simulink subsystem "PvtSubSys_HMI"  (R2020b)
settings: Solver=VariableStepAuto  StartTime=0.0  StopTime=10.0  RelTol=1e-3
undefined symbols (not defined in the file): P_HMI_LDW_LKAWarnTime, P_HMI_ObjectTypeFilter, P_HMI_WarnFormLDWReq
libraries: simulink x212, TrueDurationTime x6
(part 1 of 8)
settings Model: Creator=GW00133806  LastModifiedBy=GW00201299

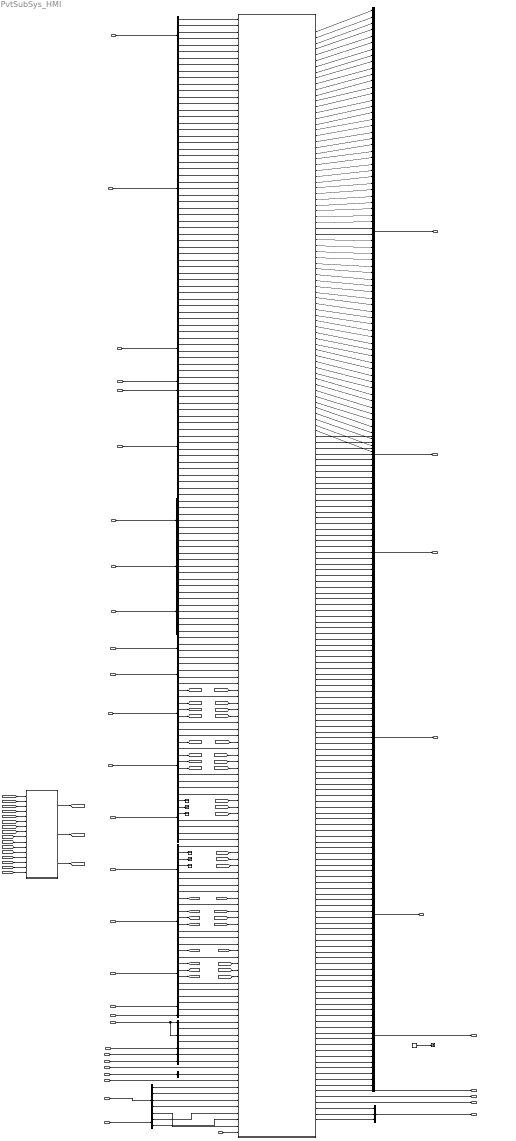
== system PvtSubSys_HMI ==
  note: HMI变更历史
      | Author:XTY
      | Version:HMI_V1.0
      | Data:2020/9/18
      | Description:
      | 可删除信号：
      |              输入：LONC_ACC_TakeOverReq；
      |                         LONC_IntelligentCurveActive；
      |              输出：Longctrl_HCUTrqReq_DVR；
      |                         ACC_TakeOverReq
      |                         Longctrl_HCUTrqReqActive_DVR
      |                         IntelligentCurveAct
      |
      | Data:2020/10/31
      | Description:
      | IFC_Signal模块：
      |                （1）增加了ELK状态显示策略
      |                （2）增加了ESS状态显示策略
      |
      | Data:2020/11/03
      | Description:
      | IFC_Signal模块：
      |                (1)增加了ELK和LCK/LKA互动关系逻辑；
      | 修正LSSErrSts逻辑；
      |                (2)增加了LSSSwt总开关逻辑；只有在LSSSwt打
      | 开的情况下，才能在3L功能任选其一；
      |                (3)增加了LCKIESts信号；方便HUT开关逻辑编写；
      |                                                                           ——2020/11/03
      |
      | Data:2020/11/05
      | Description:
      | HWA/ACC/TJA_Signal模块：
      | 1）临时增加了HWA的退出报警；
      | 11/11:
      | 增加了ACC/TJA/HWA文字提示的信号延时发送3s；
      |
      | Data:2020/11/13
      | Description:
      | （1）LDW_LKAWarn该信号接地
      | （2）释放AES输出信号：
      |           AESResp；AESSts；AESErrSts; AESintervention
      | （3）连上ACC_TakeOver；by hu；
      |
      | 2020/11/14
      | 1)ACC/TJA/HWA文字提醒调整；
      | 2)增加HMI模块的counter；
      |
      | 2020/11/19
      | 1)ACC目标显示梳理；
      | 2)HWAWarning时不报HandsOffWarning；
      |
      | 2020/11/23
      | 1)删除ACC_DataRecReq；
      | 2)HWAWarning，HandsOffWarning，DriverSts三者交互逻辑调整。
      |
      | 2020/11/30
      | （1） 增加了L1blsLineExist/ R1blsLineExist 两个信号；
      | 用来计算IFC_LaneCurve；
      | （2）关联TJAState与LSSIntervention；
      | （3）关联LSS_WarnFormSwtReq与LSSIntervention；
      | （4）增加LSSSwtReq 信号的“软开关”；修改横向功能
      | 输出；
      | （5）增加了LDW_LKAWarn信号输出
      | （6）增加了F_LBblsLineExist和F_RBblsLineExist两条
      | 边界有效性信号，用于输出计算仪表车道线信息；
      |
      | 2020/12/02
      | （1）IFCvibrationwarning信号关联LSSInTervention信号
      | only reminder coding值；
      | （2）关联TJAState与LSSIntervention及其横向状态；
      |
      | 2020/12/03
      | （1）添加了LCKSwtReq 信号；
      | （2）添加了标定量P_HMI_LDW_LKAWarnTime；
      | (3)连上ACC目标p4和p5的有效性和类型；
      |
      | 2020/12/11
      | (1)适配NOA新架构；
      | 2020/12/16
      | (1)再次适配NOA新架构，基于新EHR；
      |
      | 2020/12/22
      | 1、基于PLAN和LONG模块更新的架构调整HMI；
      | 2020/12/23
      | 增加distbar输出；
      |
      | 2020.12.29
      | 修改ACC起步提醒信号的发送，输入暂用CCTextDisp，待接口更新；
      | 2021.1.6
      | HWA转向灯请求输出；
      | 2021.1.14
      | 道线的C2,C3增加gain，参考仪表显示文档；
      | 2021.1.21
      | 修改ACC目标显示坐标系，左负右正。
      | 2021.1.27
      | ACC目标HeadingAngle输出单位修改；
      | DrvrSts修改；
      | DriverOffDisp修改；
      | 2021.2.1
      | HMI升级DBC4.1输入接口；
      | 2021.2.3
      | LSSIntervention与TJA对应状态输出修改；
      | 目标显示修改heading修改；
      | fu_type连接；
      | 2021.2.5
      | 道线长度增加12个信号输出；
      | ACCFtSts修改；
      |
      | 2021.2.17
      | 各个线C0的初始值修改；
      | 2021.2.20
      | 增加NOH相关ACC_FD3报文信号；
      | 2021.2.22
      | LCK和ELK和ESS的Error修改；
      | 接口变更增加ACCFD3；
      | HWA_LaneChangeReq修改；
      | 2021.2.25
      | HWA_LaneChangeReq修改。
      | 2021.3.2
      | RoadEdge显示输出修改；
      | 2021.3.4
      | ACC_FD2的ACC_RlvTgtDy顺序连错修改；
      | 2021.3.5
      | 目标HeadingAngle都给0；Type滤波一秒；
      | 2021.3.12
      | 目标HeadingAngle修改；LCK显示开关修改；ACC_CRInterface修改；
      | 2021.3.13-李超
      | HWA_LaneChangeReq关联HWAsts
      | 2021.3.19
      | 道线平移
      | 2021.3.24
      | Lane_Change关联Lane_ChangeReq；
      | 2021.3.25
      | Longctrl_ModSts不发failure；
      | 2021.3.26
      | ACC_DrvrOffDisp最短发3s；
      | 2021.3.27
      | 修改TJA激活但LCK开关没开时，LCKIE激活但公CAN信号不发的问题；
      | 2021.3.30
      | LongCtrl_ModSts输出修改，增加跟停后ACC故障的EPB接管逻辑；
      | 2021.4.6
      | 横向功能报警时除LDW功能外其余功能均取消方向盘震动需求，并由标定量P_HMI_WarnFormLDWReq
      | 来进行开关。（0：LDW/LKA/LCK/ELK均可方向盘震动1：仅LDW可）
      | 2021.4.8
      | HMI车道线显示修改解决
      | （1）Line01、Line02的A2系数错误导致的线交叉问题
      | （2）线有效性判断错误导致的两侧均为边界时A1/A2/A3的系数均为0的问题
  VSM_LON_CTRL : Inport  OutDataTypeStr=Bus: VSM_LON_CTRL_BUS  PortDimensions=1  BusOutputAsStruct=on
  VSM_HMI : Inport  Port=2  OutDataTypeStr=Bus: VSM_HMI_BUS  PortDimensions=1  BusOutputAsStruct=on
  HMI_VCAN_HUT : Inport  Port=3  OutDataTypeStr=Bus: VCAN_HUT_MSG_BUS  PortDimensions=1  BusOutputAsStruct=on
  DMON_SENS_ERR : Inport  Port=4  OutDataTypeStr=Bus: DMON_SENS_ERR_BUS  PortDimensions=1  BusOutputAsStruct=on
  PLAN_HMI_BUS : Inport  Port=5  OutDataTypeStr=Bus: PLAN_HMI_BUS  PortDimensions=1  BusOutputAsStruct=on
  TOS_ACCP0 : Inport  Port=6  OutDataTypeStr=Bus: TOS_ACCP0_BUS  PortDimensions=1  BusOutputAsStruct=on
  TOS_ACCP1 : Inport  Port=7  OutDataTypeStr=Bus: TOS_ACCP1_BUS  PortDimensions=1  BusOutputAsStruct=on
  TOS_ACCP2 : Inport  Port=8  OutDataTypeStr=Bus: TOS_ACCP2_BUS  PortDimensions=1  BusOutputAsStruct=on
  TOS_ACCP3 : Inport  Port=9  OutDataTypeStr=Bus: TOS_ACCP3_BUS  PortDimensions=1  BusOutputAsStruct=on
  TOS_ACCP4 : Inport  Port=10  OutDataTypeStr=Bus: TOS_ACCP4_BUS  PortDimensions=1  BusOutputAsStruct=on
  TOS_ACCP5 : Inport  Port=11  OutDataTypeStr=Bus: TOS_ACCP5_BUS  PortDimensions=1  BusOutputAsStruct=on
  RFM_LINE_L1 : Inport  Port=12  OutDataTypeStr=Bus: RFM_LINE_BUS  PortDimensions=1  BusOutputAsStruct=on
  RFM_LINE_R1 : Inport  Port=13  OutDataTypeStr=Bus: RFM_LINE_BUS  PortDimensions=1  BusOutputAsStruct=on
  RFM_LINE_L2 : Inport  Port=14  OutDataTypeStr=Bus: RFM_LINE_BUS  PortDimensions=1  BusOutputAsStruct=on
  RFM_LINE_R2 : Inport  Port=15  OutDataTypeStr=Bus: RFM_LINE_BUS  PortDimensions=1  BusOutputAsStruct=on
  RFM_LINE_LB : Inport  Port=16  OutDataTypeStr=Bus: RFM_LINE_BUS  PortDimensions=1  BusOutputAsStruct=on
  RFM_LINE_RB : Inport  Port=17  OutDataTypeStr=Bus: RFM_LINE_BUS  PortDimensions=1  BusOutputAsStruct=on
  EHRV2_ROAD_INFO : Inport  Port=18  OutDataTypeStr=Bus: EHRV2_ROAD_INFO_BUS  PortDimensions=1  BusOutputAsStruct=on
  RFM_ROAD : Inport  Port=19  OutDataTypeStr=Bus: RFM_ROAD_BUS  PortDimensions=1  BusOutputAsStruct=on
  RFM_INTERSEC_ALERT : Inport  Port=20  OutDataTypeStr=Bus: RFM_INTERSEC_ALERT_BUS  PortDimensions=1  BusOutputAsStruct=on
  EHRV2_HutHandshake : Inport  Port=21  OutDataTypeStr=uint8  PortDimensions=1  BusOutputAsStruct=on
  EHRV2_HDR : Inport  Port=22  OutDataTypeStr=Bus: EHRV2_HDR_BUS  PortDimensions=1  BusOutputAsStruct=on
  DriverSts : Inport  Port=23  OutDataTypeStr=uint8  PortDimensions=1  BusOutputAsStruct=on
  AEB_BRK_INFO : Inport  Port=24  OutDataTypeStr=Bus: AEB_BRK_INFO_BUS  PortDimensions=1  BusOutputAsStruct=on
  AEB_IPHUT_INFO : Inport  Port=25  OutDataTypeStr=Bus: AEB_IPHUT_INFO_BUS  PortDimensions=1  BusOutputAsStruct=on
  RFM_TSR : Inport  Port=26  OutDataTypeStr=Bus: RFM_TSR_BUS  PortDimensions=1  BusOutputAsStruct=on
  LONC_CTRL_OUT : Inport  Port=27  OutDataTypeStr=Bus: LONC_CTRL_OUT_BUS  PortDimensions=1  BusOutputAsStruct=on
  standstill : Inport  Port=28
  Bus Creator : BusCreator  Inputs=ACC_ModDisp,TJA_ICA_ModDisp,HWA_ModDisp,ACC_InterSysInfoDisp,TJA_ICA_InterSysInfoDisp,HWA_InterSysInfoDisp,CruCha_ModDisp,CruChar_InterSysInfoDisp,ALCResp,HWAResp,ISL_Resp,ICA_HandsOffResp,HWAwarning,ACCTimeGapSet,ACCSpdSetValue,TJA_ACCSelSts,ACCTakeOverReq,ACC_FctSts,ACC_EgoStatus,Longctrl_HazActv,ADAS_DriverInloop_Monitor,HWASnvtySetResp,HWA_Lane_ChangeReq,HWA_LaneChange,ACC_ObjDetecte,ACC_RlvTgtDetn,ACC_PotentialTgtDetn,ACC_PotentialTgtTyp,ACC_PotentialTgtDx,ACC_PotentialTgtDy,ACC_LeTargrtDection,ACC_LeTgtTyp,ACC_LeTgtDx,ACC_LeTgtDy,ACC_RiTargrtDetn,ACC_RiTgtTyp,ACC_RiTgtDx,ACC_RiTgtDy,ISLInterSysInfoDisp,Longctrl_DrvOFF_Req_DVR,Longctrl_ModSts_DVR,Longctrl_ParkShiftReq_DVR,ACC_RlvTgtTyp,ACC_RlvTgtDx,ACC_RlvTgtDy,Longctrl_HCUTrqReq_DVR,ALC_InterSysInfoDisp,Request_driveoff,Longctrl_VehHldReq_DVR,Longctrl_HCUTrqReqActive_DVR,IntelligentCurveAct,ACC_RlvTgtfusion,ACC_RlvTgtHeading,ACC_LeTgtfusion,ACC_LeTgtHeading,ACC_RiTgtfusion,ACC_RiTgtHeading,ACC_PotentialTgtfusion,ACC_PotentialTgtHeading,ACC_LeTgt_02_Dy,ACC_LeTgt_02_Dx,ACC_LeTgt_02_Typ,ACC_LeTargrt_02_Detn,ACC_RiTargrt_02_Detn,ACC_RiTgt_02_Dy,ACC_RiTgt_02_Dx,ACC_RiTgt_02_Typ,ACCTgtObjBarDisp,ACCLeTgtObjBarDisp,ACCRiTgtObjBarDisp
  Bus Creator1 : BusCreator  Inputs=7
  Bus Creator2 : BusCreator  Inputs=ACCTgtObjDx,ACCTgtObjDy,ACCTgtObjObstcl,ACCTgtObjExist,ACCTgtObjVy,ACCTgtObjVx,ACCTgtObjAx,ACCTgtObjAy,ACCTgtObjState,ACCTgtObjVideoCfmd,ACCTgtObjCntAlive,Handsoff_Detd,DrvgOnHiWay,RoadCrvt,SpdLimitDst,RoadCrvtFar,RampDst,SpdLimit,CurveDst,NavSpdLimUnit,TunnelDst,Drvg_OnRiLane,BrdgDst,ACC_SOSReq,Map_DataValid,DrvrSts,ACCTgtObjID
  Bus Creator3 : BusCreator  Inputs=37
  Bus Creator4 : BusCreator  Inputs=24
  Bus Creator5 : BusCreator  Inputs=18
  Bus Creator6 : BusCreator  Inputs=3
  Bus Selector : BusSelector  OutputSignals=TJASts,HWASts,HWAActive,ACC_HazActv,ACC_ModeDisp,ACC_ParkShiftReq,TJA_ModeDisp,HWA_ModeDisp,HWASlowRetreat_b,CruiseChauffeur_ModeDisp,ACCTextDisp,TJATextDisp,CCTextDisp,HWATextDisp,LCKSts,HandsOffWarningLevel,LDWSts,LKASts,LKAWarning,ELKSts,LCKIESts,ACC_ISLResp,ISL_InterSysInfoDisp,ISLActive,ALC_Resp,HWA_SnvtySet_Resp,HWA_Resp,ICA_HandsOffSwtResp,TJA_ACC_SelSts,HWA_LaneChangeReq,HWA_Warning,HandsOffDetd,LSS_WarnFormSwtResp,DriverInloop_Monitor,ACC_SOS_Req,LaneAvailability,TJA_FollowSts,ESSSts,AESSts,HWA_TurnLightReq,ACC_DrvrOffDisp
  Bus Selector1 : BusSelector  OutputSignals=Longctrl_Decel_Req
  Bus Selector10 : BusSelector  OutputSignals=dyP5,dxP5,ObjTypeP5,targetExistP5
  Bus Selector{11..12,15..16} (4 alike) : BusSelector  OutputSignals=bIsLineExist,dC0V,dC1V,dC2V,dC3V,eLineType,dDisStart,dDisFront
  Bus Selector13 : BusSelector  OutputSignals=dC0V,dC1V,dC2V,dC3V,eLineType,dDisStart,dDisFront,bIsLineExist
  Bus Selector14 : BusSelector  OutputSignals=dC0V,dC1V,dC2V,dC3V,eLineType,dDisStart,dDisFront,bIsLineExist
  Bus Selector17 : BusSelector  OutputSignals=i_func_road_class
  Bus Selector18 : BusSelector  OutputSignals=i_road_curvature_far_distance,i_road_curvature,i_road_curvature_far
  Bus Selector19 : BusSelector  OutputSignals=TSR_Sign_Long_Distance
  Bus Selector2 : BusSelector  OutputSignals=IDP0,dxP0,vxRelP0,ACCTgtObjVy,axAbsGroundP0,targetExistP0,fu_typeP0,ObjMovingStateP0,Object_Orientation,ObjTypeP0,ObjDYP0,ACCTgtObjObstcl,ACCTgtObjAy,ACCTgtObjCntAlive,ACCTgtObjExist,P0HeadingAngle
  Bus Selector20 : BusSelector  OutputSignals=FCW_Warn
  Bus Selector21 : BusSelector  OutputSignals=AEB_TgtDecel_Req
  Bus Selector22 : BusSelector  OutputSignals=f_toll_distance,f_bridge_distance
  Bus Selector23 : BusSelector  OutputSignals=f_start_distance
  Bus Selector24 : BusSelector  OutputSignals=MapDataValid
  Bus Selector25 : BusSelector  OutputSignals=tor,ACC_TgtObjBarDisp,ACC_LeTgtObjBarDisp,ACC_RiTgtObjBarDisp,IntelligentCurveActive
  Bus Selector26 : BusSelector  OutputSignals=LKASwtReq,LCKSwtReq
  Bus Selector3 : BusSelector  OutputSignals=ACCSts,ACC_SpdSetValue,ACC_TimeGapSet_HMI,ACC_DrvOffReq,vSetBelowMin,HWAAccControlSts
  Bus Selector4 : BusSelector  OutputSignals=LSSSwtReq,ESS_PedSwtReq,ESS_VehSwtReq,AESSwtReq,IFC_SnvtySet,ADAS_Posn_CurLane,NavSpdLimValue,NavSpdLimUnit_HUT
  Bus Selector5 : BusSelector  OutputSignals=FCam_CalibrationSts,FCam_BlockageSts
  Bus Selector6 : BusSelector  OutputSignals=IDP1,dxP1,targetExistP1,fu_typeP1,ObjTypeP1,ObjDYP1,P1HeadingAngle
  Bus Selector7 : BusSelector  OutputSignals=IDP2,dxP2,targetExistP2,fu_typeP2,ObjTypeP2,ObjDYP2,P2HeadingAngle
  Bus Selector8 : BusSelector  OutputSignals=IDP3,dxP3,targetExistP3,fu_typeP3,ObjTypeP3,ObjDYP3,P3HeadingAngle
  Bus Selector9 : BusSelector  OutputSignals=dyP4,dxP4,ObjTypeP4,targetExistP4
  Counter Limited : simulink/Sources/Counter Limited  uplimit=255  tsamp=-1
  HMI2.12 : Subsystem
  HMI_VCAN_HUT_1 : InportShadow  Port=3  OutDataTypeStr=Bus: VCAN_HUT_MSG_BUS  PortDimensions=1  BusOutputAsStruct=on
  MATLAB Function1 : MATLAB Function  TreatAsAtomicUnit=on
  Terminator{,1..6} (7 alike) : Terminator
  HMI_IFC_FD2 : Outport  OutDataTypeStr=Bus: HMI_IFC_FD2_BUS  PortDimensions=1  BusOutputAsStruct=on
  HMI_IFCVibrationWarning : Outport  Port=2  OutDataTypeStr=uint8  PortDimensions=1  BusOutputAsStruct=on
  HMI_ESSErrSts : Outport  Port=3  OutDataTypeStr=boolean  BusOutputAsStruct=on
  HMI_AESErrSts : Outport  Port=4  OutDataTypeStr=boolean  BusOutputAsStruct=on
  HMI_ACC_FD2 : Outport  Port=5  OutDataTypeStr=Bus: HMI_ACC_FD2_BUS  PortDimensions=1  BusOutputAsStruct=on
  HMI_ACC_FD4 : Outport  Port=6  OutDataTypeStr=Bus: HMI_ACC_FD4_BUS  PortDimensions=1  BusOutputAsStruct=on
  HMI_ACC_FD1 : Outport  Port=7  OutDataTypeStr=Bus: HMI_ACC_FD1_BUS  PortDimensions=1  BusOutputAsStruct=on
  HMI_IFC_FD5 : Outport  Port=8  OutDataTypeStr=Bus: HMI_IFC_FD5_BUS  PortDimensions=1  BusOutputAsStruct=on
  HMI_IFC_FD6 : Outport  Port=9  OutDataTypeStr=Bus: HMI_IFC_FD6_BUS  PortDimensions=1  BusOutputAsStruct=on
  HMI_IFC_FD3 : Outport  Port=10  OutDataTypeStr=Bus: HMI_IFC_FD3_BUS  PortDimensions=1  BusOutputAsStruct=on
  wires:
  Bus Selector4/8 -> HMI2.12/55(NavSpdLimUnit_HUT)  "<NavSpdLimUnit_HUT>"
  HMI2.12/42(Longctrl_ParkShiftReq_DVR) -> Bus Creator/42
  HMI2.12/167(IFC_Line02_HeadingAngle) -> Bus Creator5/2
  LONC_CTRL_OUT/1 -> Bus Selector1/1
  Bus Creator2/1 -> HMI_ACC_FD4/1
  HMI2.12/17(ACC_TakeOverReq) -> Bus Creator/17
  HMI2.12/174(IFC_Line02_DxStart) -> Bus Creator5/9
  Bus Selector16/2 -> HMI2.12/145(F_RBdC0V)  "<dC0V>"
  HMI2.12/175(IFC_Line02_DxEnd) -> Bus Creator5/10
  Bus Selector7/4 -> HMI2.12/85(fu_typeP2)  "<fu_typeP2>"
  HMI2.12/2(TJA_ICA_ModDisp) -> Bus Creator/2
  Bus Selector/26 -> HMI2.12/32(HWA_SnvtySet_Resp)  "<HWA_SnvtySet_Resp>"
  PLAN_HMI_BUS/1 -> Bus Selector25/1
  HMI2.12/164(IFC_Roadedge02_CurvChange) -> Bus Creator4/23
  Bus Selector7/2 -> HMI2.12/83(dxP2)  "<dxP2>"
  HMI2.12/111(IntelligentEvaResp) -> Bus Creator3/7
  HMI2.12/72(Longctrl_ModSts) -> Bus Creator1/2
  HMI2.12/76(ACC_CRInterface) -> Bus Creator1/6
  Bus Selector25/4 -> HMI2.12/168(ACC_RiTgtObjBarDisp)  "<ACC_RiTgtObjBarDisp>"
  HMI2.12/112(LSSFuncSts) -> Bus Creator3/8
  Bus Selector/1 -> HMI2.12/7(TJASts)  "<TJASts>"
  Bus Selector2/7 -> HMI2.12/65(fu_typeP0)  "<fu_typeP0>"
  HMI2.12/43(ACC_RlvTgtTyp) -> Bus Creator/43
  HMI2.12/91(RoadCrvt) -> Bus Creator2/14
  Bus Selector/4 -> HMI2.12/10(ACC_HazActv)  "<ACC_HazActv>"
  Bus Selector/23 -> HMI2.12/29(ISL_InterSysInfoDisp)  "<ISL_InterSysInfoDisp>"
  Bus Selector25/1 -> HMI2.12/165(Long_ACCTakeoverReq)  "<tor>"
  Bus Selector2/12 -> HMI2.12/70(ACCTgtObjObstcl)  "<ACCTgtObjObstcl>"
  TOS_ACCP1/1 -> Bus Selector6/1
  HMI2.12/148(IFC_Line02_CurvChange) -> Bus Creator4/7
  Bus Selector12/7 -> HMI2.12/118(R1dDisStart)  "<dDisStart>"
  HMI2.12/168(IFC_Line03_HeadingAngle) -> Bus Creator5/3
  Bus Selector9/1 -> HMI2.12/96(dyP4)  "<dyP4>"
  Bus Selector/18 -> HMI2.12/24(LKAState)  "<LKASts>"
  HMI2.12/176(IFC_Line03_DxStart) -> Bus Creator5/11
  HMI2.12/126(IFC_LeLaneTyp) -> Bus Creator3/22
  HMI2.12/156(IFC_Line04_CurvChange) -> Bus Creator4/15
  Bus Selector/27 -> HMI2.12/33(HWA_Resp)  "<HWA_Resp>"
  Bus Selector11/8 -> HMI2.12/111(L1dDisFront)  "<dDisFront>"
  DMON_SENS_ERR/1 -> Bus Selector5/1
  HMI2.12/44(ACC_RlvTgtDx) -> Bus Creator/44
  Bus Selector8/7 -> HMI2.12/95(P3HeadingAngle)  "<P3HeadingAngle>"
  HMI2.12/70(ACCRiTgtObjBarDisp) -> Bus Creator/70
  HMI2.12/135(AESintervention) -> Bus Creator3/31
  HMI2.12/188(IDC_L2_TurnLightReq) -> Bus Creator6/2
  HMI2.12/37(ACC_RiTgtDx) -> Bus Creator/37
  HMI2.12/20(Longctrl_HazActv) -> Bus Creator/20
  HMI2.12/98(TunnelDst) -> Bus Creator2/21
  HMI2.12/14(ACCTimeGapSet) -> Bus Creator/14
  HMI2.12/101(ACC_SOSReq) -> Bus Creator2/24
  Bus Selector/29 -> HMI2.12/35(TJA_ACC_SelSts)  "<TJA_ACC_SelSts>"
  Bus Selector9/2 -> HMI2.12/97(dxP4)  "<dxP4>"
  Bus Selector10/1 -> HMI2.12/100(dyP5)  "<dyP5>"
  Bus Selector/40 -> HMI2.12/46(HWA_TurnLightReq)  "<HWA_TurnLightReq>"
  Bus Selector14/1 -> HMI2.12/128(R2dC0V)  "<dC0V>"
  HMI2.12/184(IFCVibrationWarning) -> HMI_IFCVibrationWarning/1
  Bus Creator5/1 -> HMI_IFC_FD6/1
  Bus Selector2/15 -> HMI2.12/73(ACCTgtObjExist)  "<ACCTgtObjExist>"
  HMI2.12/47(ALC_InterSysInfoDisp) -> Bus Creator/47
  Bus Selector8/3 -> HMI2.12/91(targetExistP3)  "<targetExistP3>"
  Bus Selector7/1 -> HMI2.12/82(IDP2)  "<IDP2>"
  RFM_LINE_L2/1 -> Bus Selector13/1
  Bus Selector2/2 -> HMI2.12/60(dxP0)  "<dxP0>"
  Bus Selector7/3 -> HMI2.12/84(targetExistP2)  "<targetExistP2>"
  Bus Selector19/1 -> HMI2.12/161(TSR_Sign_Long_Distance)  "<TSR_Sign_Long_Distance>"
  HMI2.12/84(ACCTgtObjAx) -> Bus Creator2/7
  HMI2.12/130(IFC_LaneCurve) -> Bus Creator3/26
  Bus Selector10/3 -> HMI2.12/102(ObjTypeP5)  "<ObjTypeP5>"
  HMI2.12/127(IFC_RiLaneTyp) -> Bus Creator3/23
  HMI2.12/9(ALCResp) -> Bus Creator/9
  HMI2.12/125(TJAFollowSts) -> Bus Creator3/21
  HMI2.12/159(IFC_Roadedge01_Curv) -> Bus Creator4/18
  HMI2.12/12(ICA_HandsOffResp) -> Bus Creator/12
  Bus Selector/15 -> HMI2.12/21(LCKSts)  "<LCKSts>"
  RFM_INTERSEC_ALERT/1 -> Bus Selector23/1
  Bus Selector10/2 -> HMI2.12/101(dxP5)  "<dxP5>"
  Bus Creator/1 -> HMI_ACC_FD2/1
  Bus Selector14/6 -> HMI2.12/133(R2dDisStart)  "<dDisStart>"
  Bus Selector8/1 -> HMI2.12/89(IDP3)  "<IDP3>"
  Bus Selector/16 -> HMI2.12/22(HandsOffWarningLevel)  "<HandsOffWarningLevel>"
  HMI2.12/85(ACC_TgtObjAy) -> Bus Creator2/8
  HMI2.12/140(AES_Sts) -> Bus Creator3/36
  HMI_VCAN_HUT_1/1 -> Bus Selector26/1
  HMI2.12/179(IFC_Line04_DxEnd) -> Bus Creator5/14
  HMI2.12/13(HWAwarning) -> Bus Creator/13
  TOS_ACCP0/1 -> Bus Selector2/1
  Bus Selector16/8 -> HMI2.12/151(E2dDisStart)  "<dDisFront>"
  Bus Selector1/1 -> HMI2.12/58(ACC_Decel_Req)  "<Longctrl_Decel_Req>"
  HMI2.12/52(ACC_RlvTgtfusion) -> Bus Creator/52
  HMI2.12/28(ACC_PotentialTgtTyp) -> Bus Creator/28
  HMI2.12/181(IFC_Roadedge01_DxEnd) -> Bus Creator5/16
  HMI2.12/113(LSSErrSts) -> Bus Creator3/9
  HMI2.12/68(ACCTgtObjBarDisp) -> Bus Creator/68
  HMI2.12/8(CruChar_InterSysInfoDisp) -> Bus Creator/8
  HMI2.12/107(ELKResp) -> Bus Creator3/3
  Bus Selector/25 -> HMI2.12/31(ALC_Resp)  "<ALC_Resp>"
  Bus Creator3/1 -> HMI_IFC_FD2/1
  HMI2.12/157(IFC_Line04_Type) -> Bus Creator4/16
  Bus Selector14/7 -> HMI2.12/134(R2dDisFront)  "<dDisFront>"
  HMI2.12/104(ACCTgtObjID) -> Bus Creator2/27
  Bus Selector13/6 -> HMI2.12/125(L2dDisStart)  "<dDisStart>"
  HMI2.12/81(ACC_TgtObjExist) -> Bus Creator2/4
  Bus Selector/21 -> HMI2.12/27(LCKIESts)  "<LCKIESts>"
  Bus Selector13/7 -> HMI2.12/126(L2dDisFront)  "<dDisFront>"
  Bus Selector15/7 -> HMI2.12/142(E1dDisStart)  "<dDisStart>"
  HMI2.12/32(ACC_LeTgtTyp) -> Bus Creator/32
  VSM_LON_CTRL/1 -> Bus Selector3/1
  VSM_HMI/1 -> Bus Selector/1
  Bus Selector15/8 -> HMI2.12/143(E1dDisFront)  "<dDisFront>"
  Bus Selector5/1 -> HMI2.12/56(IFC_CalibrationSts)  "<FCam_CalibrationSts>"
  Bus Selector2/13 -> HMI2.12/71(ACCTgtObjAy)  "<ACCTgtObjAy>"
  HMI2.12/132(IFC_RiLane_dy) -> Bus Creator3/28
  HMI2.12/30(ACC_PotentialTgtDy) -> Bus Creator/30
  HMI2.12/49(Longctrl_VehHldReq_DVR) -> Bus Creator/49
  HMI2.12/51(IntelligentCurveAct) -> Bus Creator/51
  HMI2.12/117(ESS_PedResp) -> Bus Creator3/13
  HMI2.12/90(DrvgOnHiWay) -> Bus Creator2/13
  HMI2.12/19(ACC_EgoStatus) -> Bus Creator/19
  Bus Selector2/8 -> HMI2.12/66(ObjMovingStateP0)  "<ObjMovingStateP0>"
  RFM_LINE_LB/1 -> Bus Selector15/1
  HMI2.12/1(ACC_ModDisp) -> Bus Creator/1
  HMI2.12/73(Longctrl_ParkShiftReq) -> Bus Creator1/3
  RFM_LINE_RB/1 -> Bus Selector16/1
  Bus Selector12/2 -> HMI2.12/113(R1dC0V)  "<dC0V>"
  HMI2.12/145(IFC_Line01_Type) -> Bus Creator4/4
  Bus Selector24/1 -> HMI2.12/163(MapDataValid)  "<MapDataValid>"
  HMI2.12/80(ACC_TgtObjObstcl) -> Bus Creator2/3
  Bus Selector/33 -> HMI2.12/39(LSS_WarnFormSwtResp)  "<LSS_WarnFormSwtResp>"
  HMI2.12/33(ACC_LeTgtDx) -> Bus Creator/33
  HMI2.12/3(HWA_ModDisp) -> Bus Creator/3
  HMI2.12/173(IFC_Line01_DxEnd) -> Bus Creator5/8
  Bus Selector/31 -> HMI2.12/37(HWA_Warning)  "<HWA_Warning>"
  HMI2.12/114(LSSResp) -> Bus Creator3/10
  Bus Selector16/7 -> HMI2.12/150(E2dDisFront)  "<dDisStart>"
  HMI2.12/16(TJA_ACCSelSts) -> Bus Creator/16
  HMI_VCAN_HUT/1 -> Bus Selector4/1
  Bus Selector11/7 -> HMI2.12/110(L1dDisStart)  "<dDisStart>"
  Bus Selector/14 -> HMI2.12/20(HWATextDisp)  "<HWATextDisp>"
  Bus Selector/28 -> HMI2.12/34(ICA_HandsOffSwtResp)  "<ICA_HandsOffSwtResp>"
  HMI2.12/65(ACC_RiTgt_02_Dy) -> Bus Creator/65
  Bus Selector/2 -> HMI2.12/8(HWASts)  "<HWASts>"
  HMI2.12/178(IFC_Line04_DxStart) -> Bus Creator5/13
  HMI2.12/171(IFC_Roadedge02_HeadingAngle) -> Bus Creator5/6
  Bus Selector12/8 -> HMI2.12/119(R1dDisFront)  "<dDisFront>"
  HMI2.12/138(IntelligentEvaActSts) -> Bus Creator3/34
  HMI2.12/133(IFC_NextLeLane_dy) -> Bus Creator3/29
  HMI2.12/102(Map_DataValid) -> Bus Creator2/25
  HMI2.12/35(ACC_RiTargrtDetn) -> Bus Creator/35
  HMI2.12/61(ACC_LeTgt_02_Dx) -> Bus Creator/61
  RFM_TSR/1 -> Bus Selector19/1
  Bus Selector12/6 -> HMI2.12/117(R1enLineType)  "<eLineType>"
  HMI2.12/39(ISLInterSysInfoDisp) -> Bus Creator/39
  HMI2.12/74(ActualTargetSpeed) -> Bus Creator1/4
  HMI2.12/86(ACCTgtObjState) -> Bus Creator2/9
  HMI2.12/95(SpdLimit) -> Bus Creator2/18
  Bus Selector/7 -> HMI2.12/13(TJA_ModeDisp)  "<TJA_ModeDisp>"
  Bus Selector/3 -> HMI2.12/9(HWAActive)  "<HWAActive>"
  HMI2.12/69(ACCLeTgtObjBarDisp) -> Bus Creator/69
  HMI2.12/155(IFC_Line04_Curv) -> Bus Creator4/14
  EHRV2_ROAD_INFO/1 -> Bus Selector17/1, Bus Selector18/1
  HMI2.12/120(IFC_LaneAvailability) -> Bus Creator3/16
  Bus Selector/11 -> HMI2.12/17(ACCTextDisp)  "<ACCTextDisp>"
  HMI2.12/94(RampDst) -> Bus Creator2/17
  HMI2.12/182(IFC_Roadedge02_DxStart) -> Bus Creator5/17
  HMI2.12/177(IFC_Line03_DxEnd) -> Bus Creator5/12
  Bus Selector11/2 -> HMI2.12/105(L1dC0V)  "<dC0V>"
  EHRV2_HutHandshake/1 -> HMI2.12/164(IFCHUTInterface)
  Bus Selector13/5 -> HMI2.12/124(L2enLineType)  "<eLineType>"
  HMI2.12/124(CameraBlockageSts) -> Bus Creator3/20
  Bus Selector/12 -> HMI2.12/18(TJATextDisp)  "<TJATextDisp>"
  HMI2.12/180(IFC_Roadedge01_DxStart) -> Bus Creator5/15
  Bus Selector/8 -> HMI2.12/14(HWA_ModeDisp)  "<HWA_ModeDisp>"
  HMI2.12/183(IFC_Roadedge02_DxEnd) -> Bus Creator5/18
  HMI2.12/106(LSSWarnFormResp) -> Bus Creator3/2
  Bus Selector6/2 -> HMI2.12/76(dxP1)  "<dxP1>"
  Bus Selector/5 -> HMI2.12/11(ACC_ModeDisp)  "<ACC_ModeDisp>"
  HMI2.12/18(ACC_FctSts) -> Bus Creator/18
  Bus Selector4/1 -> HMI2.12/48(LSSSwtReq)  "<LSSSwtReq>"
  HMI2.12/134(IFC_NextRiLane_dy) -> Bus Creator3/30
  Bus Selector18/2 -> HMI2.12/157(RoadCurvature)  "<i_road_curvature>"
  Bus Selector25/2 -> HMI2.12/166(ACC_TgtObjBarDisp)  "<ACC_TgtObjBarDisp>"
  Bus Selector14/5 -> HMI2.12/132(R2enLineType)  "<eLineType>"
  HMI2.12/57(ACC_RiTgtHeading) -> Bus Creator/57
  Bus Selector25/3 -> HMI2.12/167(ACC_LeTgtObjBarDisp)  "<ACC_LeTgtObjBarDisp>"
  HMI2.12/92(SpdLimitDst) -> Bus Creator2/15
  HMI2.12/163(IFC_Roadedge02_Curv) -> Bus Creator4/22
  HMI2.12/53(ACC_RlvTgtHeading) -> Bus Creator/53
  HMI2.12/172(IFC_Line01_DxStart) -> Bus Creator5/7
  AEB_IPHUT_INFO/1 -> Bus Selector20/1
  Bus Selector/36 -> HMI2.12/42(LaneAvailability)  "<LaneAvailability>"
  RFM_LINE_R1/1 -> Bus Selector12/1
  Bus Selector/30 -> HMI2.12/36(HWA_LaneChangeReq)  "<HWA_LaneChangeReq>"
  Bus Selector6/3 -> HMI2.12/77(targetExistP1)  "<targetExistP1>"
  Bus Selector3/2 -> HMI2.12/2(ACC_SpdSetValue)  "<ACC_SpdSetValue>"
  HMI2.12/144(IFC_Line01_CurvChange) -> Bus Creator4/3
  Bus Selector20/1 -> HMI2.12/160(Inter_FCW_Warn)  "<FCW_Warn>"
  Bus Selector8/4 -> HMI2.12/92(fu_typeP3)  "<fu_typeP3>"
  Bus Creator1/1 -> HMI_ACC_FD1/1
  HMI2.12/56(ACC_RiTgtfusion) -> Bus Creator/56
  HMI2.12/118(ESS_VehResp) -> Bus Creator3/14
  Bus Selector6/6 -> HMI2.12/80(ObjDYP1)  "<ObjDYP1>"
  Bus Selector/13 -> HMI2.12/19(CCTextDisp)  "<CCTextDisp>"
  Bus Selector/6 -> HMI2.12/12(ACC_ParkShiftReq)  "<ACC_ParkShiftReq>"
  Bus Selector18/3 -> HMI2.12/158(RoadCurvatureFar)  "<i_road_curvature_far>"
  HMI2.12/154(IFC_Line04_Dy) -> Bus Creator4/13
  HMI2.12/165(IFC_Roadedge02_Type) -> Bus Creator4/24
  Bus Selector/39 -> HMI2.12/45(AESSts)  "<AESSts>"
  HMI2.12/67(ACC_RiTgt_02_Typ) -> Bus Creator/67
  Bus Selector2/1 -> HMI2.12/59(IDP0)  "<IDP0>"
  HMI2.12/151(IFC_Line03_Curv) -> Bus Creator4/10
  Bus Selector25/5 -> HMI2.12/171(IntelligentCurveActive)  "<IntelligentCurveActive>"
  HMI2.12/24(HWA_LaneChange) -> Bus Creator/24
  HMI2.12/26(ACC_RlvTgtDetn) -> Bus Creator/26
  HMI2.12/142(IFC_Line01_Dy) -> Bus Creator4/1
  Bus Selector8/6 -> HMI2.12/94(ObjDYP3)  "<ObjDYP3>"
  Bus Selector4/7 -> HMI2.12/54(NavSpdLimValue)  "<NavSpdLimValue>"
  Bus Selector/38 -> HMI2.12/44(ESSSts)  "<ESSSts>"
  Bus Selector2/9 -> HMI2.12/67(Object_Orientation)  "<Object_Orientation>"
  HMI2.12/109(LKAResp) -> Bus Creator3/5
  Bus Selector6/4 -> HMI2.12/78(fu_typeP1)  "<fu_typeP1>"
  DriverSts/1 -> HMI2.12/162(DrvrState)
  HMI2.12/116(LDW_LKAWarn) -> Bus Creator3/12
  HMI2.12/6(HWA_InterSysInfoDisp) -> Bus Creator/6
  Counter Limited/1 -> Terminator3/1  "HMI_Counter"
  Bus Selector3/3 -> HMI2.12/3(ACC_TimeGapSet)  "<ACC_TimeGapSet_HMI>"
  EHRV2_HDR/1 -> Bus Selector24/1
  HMI2.12/55(ACC_LeTgtHeading) -> Bus Creator/55
  Bus Selector/32 -> HMI2.12/38(HandsoffDetd)  "<HandsOffDetd>"
  Bus Selector16/6 -> HMI2.12/149(F_RBenLineType)  "<eLineType>"
  Bus Selector2/16 -> HMI2.12/74(P0HeadingAngle)  "<P0HeadingAngle>"
  Bus Selector/9 -> HMI2.12/15(HWASlowRetreat_b)  "<HWASlowRetreat_b>"
  HMI2.12/10(HWAResp) -> Bus Creator/10
  Bus Selector2/10 -> HMI2.12/68(ObjTypeP0)  "<ObjTypeP0>"
  HMI2.12/141(ESS_Sts) -> Bus Creator3/37
  HMI2.12/58(ACC_PotentialTgtfusion) -> Bus Creator/58
  HMI2.12/78(ACCTgtObjDx) -> Bus Creator2/1
  RFM_LINE_R2/1 -> Bus Selector14/1
  HMI2.12/11(ISL_Resp) -> Bus Creator/11
  Bus Selector7/7 -> HMI2.12/88(P2HeadingAngle)  "<P2HeadingAngle>"
  HMI2.12/87(ACCTgtObjVideoCfmd) -> Bus Creator2/10
  Bus Selector/34 -> HMI2.12/40(DriverInloop_Monitor)  "<DriverInloop_Monitor>"
  Bus Selector6/7 -> HMI2.12/81(P1HeadingAngle)  "<P1HeadingAngle>"
  Bus Selector7/5 -> HMI2.12/86(ObjTypeP2)  "<ObjTypeP2>"
  HMI2.12/31(ACC_LeTargrtDection) -> Bus Creator/31
  HMI2.12/63(ACC_LeTargrt_02_Detn) -> Bus Creator/63
  HMI2.12/15(ACCSpdSetValue) -> Bus Creator/15
  HMI2.12/75(Longctrl_VehHldReq) -> Bus Creator1/5
  TOS_ACCP3/1 -> Bus Selector8/1
  TOS_ACCP5/1 -> Bus Selector10/1
  HMI2.12/77(Longctrl_FuelCutOffPrevn) -> Bus Creator1/7
  HMI2.12/99(Drvg_OnRiLane) -> Bus Creator2/22
  HMI2.12/129(IFC_NextRiLaneTyp) -> Bus Creator3/25
  HMI2.12/146(IFC_Line02_Dy) -> Bus Creator4/5
  HMI2.12/170(IFC_Roadedge01_HeadingAngle) -> Bus Creator5/5
  Bus Selector4/6 -> HMI2.12/53(ADAS_Posn_CurLane)  "<ADAS_Posn_CurLane>"
  HMI2.12/41(Longctrl_ModSts_DVR) -> Bus Creator/41
  Bus Selector23/1 -> HMI2.12/154(RampDistance)  "<f_start_distance>"
  HMI2.12/189(IDC_L2_FWiperReq) -> Bus Creator6/3
  Bus Selector/35 -> HMI2.12/41(ACC_SOS_Req)  "<ACC_SOS_Req>"
  HMI2.12/59(ACC_PotentialTgtHeading) -> Bus Creator/59
  HMI2.12/149(IFC_Line02_Type) -> Bus Creator4/8
  HMI2.12/185(AESErrSts) -> HMI_AESErrSts/1
  Bus Selector4/5 -> HMI2.12/52(IFC_SnvtySet)  "<IFC_SnvtySet>"
  HMI2.12/40(Longctrl_DrvOFF_Req_DVR) -> Bus Creator/40
  HMI2.12/38(ACC_RiTgtDy) -> Bus Creator/38
  HMI2.12/50(Longctrl_HCUTrqReqActive_DVR) -> Bus Creator/50
  Bus Selector9/4 -> HMI2.12/99(targetExistP4)  "<targetExistP4>"
  Bus Selector15/6 -> HMI2.12/141(F_LBenLineType)  "<eLineType>"
  HMI2.12/89(Handsoff_Detd) -> Bus Creator2/12
  Bus Selector/22 -> HMI2.12/28(ACC_ISLResp)  "<ACC_ISLResp>"
  Bus Selector4/4 -> HMI2.12/51(AESSwtReq)  "<AESSwtReq>"
  HMI2.12/79(ACCTgtObjDy) -> Bus Creator2/2
  HMI2.12/152(IFC_Line03_CurvChange) -> Bus Creator4/11
  RFM_ROAD/1 -> Bus Selector22/1
  Bus Selector2/6 -> HMI2.12/64(targetExistP0)  "<targetExistP0>"
  Bus Selector18/1 -> HMI2.12/156(RoadCurvatureFarDistance)  "<i_road_curvature_far_distance>"
  HMI2.12/25(ACC_ObjDetecte) -> Bus Creator/25
  HMI2.12/150(IFC_Line03_Dy) -> Bus Creator4/9
  Bus Selector2/5 -> HMI2.12/63(axAbsGroundP0)  "<axAbsGroundP0>"
  HMI2.12/143(IFC_Line01_Curv) -> Bus Creator4/2
  HMI2.12/147(IFC_Line02_Curv) -> Bus Creator4/6
  HMI2.12/105(LSSIntervention) -> Bus Creator3/1
  HMI2.12/27(ACC_PotentialTgtDetn) -> Bus Creator/27
  Bus Selector6/1 -> HMI2.12/75(<IDP1>)  "<IDP1>"
  Bus Selector11/6 -> HMI2.12/109(L1enLineType)  "<eLineType>"
  Bus Selector10/4 -> HMI2.12/103(targetExistP5)  "<targetExistP5>"
  Bus Selector2/4 -> HMI2.12/62(ACCTgtObjVy)  "<ACCTgtObjVy>"
  HMI2.12/100(BrdgDst) -> Bus Creator2/23
  HMI2.12/97(NavSpdLimUnit) -> Bus Creator2/20
  Bus Selector9/3 -> HMI2.12/98(ObjTypeP4)  "<ObjTypeP4>"
  Bus Selector3/4 -> HMI2.12/4(ACC_DrvOffReq)  "<ACC_DrvOffReq>"
  HMI2.12/137(ELKActSts) -> Bus Creator3/33
  HMI2.12/166(IFC_Line01_HeadingAngle) -> Bus Creator5/1
  Bus Selector21/1 -> HMI2.12/159("Inter_AEB_TgtDecel_Req ")  "<AEB_TgtDecel_Req>"
  HMI2.12/158(IFC_Roadedge01_Dy) -> Bus Creator4/17
  TOS_ACCP2/1 -> Bus Selector7/1
  HMI2.12/115(ELKMainState) -> Bus Creator3/11
  Bus Selector26/2 -> HMI2.12/170(LCKSwtReq)  "<LCKSwtReq>"
  AEB_BRK_INFO/1 -> Bus Selector21/1
  HMI2.12/83(ACCTgtObjVx) -> Bus Creator2/6
  Bus Selector/10 -> HMI2.12/16(CruiseChauffeur_ModeDisp)  "<CruiseChauffeur_ModeDisp>"
  Bus Selector4/3 -> HMI2.12/50(ESS_VehSwtReq)  "<ESS_VehSwtReq>"
  Bus Selector2/3 -> HMI2.12/61(vxRelP0)  "<vxRelP0>"
  Bus Selector/20 -> HMI2.12/26(ELKSts)  "<ELKSts>"
  HMI2.12/7(CruCha_ModDisp) -> Bus Creator/7
  HMI2.12/34(ACC_LeTgtDy) -> Bus Creator/34
  Bus Selector7/6 -> HMI2.12/87(ObjDYP2)  "<ObjDYP2>"
  HMI2.12/93(RoadCrvtFar) -> Bus Creator2/16
  Bus Selector4/2 -> HMI2.12/49(ESS_PedSwtReq)  "<ESS_PedSwtReq>"
  HMI2.12/110(LDWResp) -> Bus Creator3/6
  Bus Selector3/1 -> HMI2.12/1(ACCSts)  "<ACCSts>"
  HMI2.12/162(IFC_Roadedge02_Dy) -> Bus Creator4/21
  Bus Selector17/1 -> HMI2.12/155(DrivingOnHighWay)  "<i_func_road_class>"
  HMI2.12/128(IFC_NextLeLaneTyp) -> Bus Creator3/24
  HMI2.12/103(DrvrSts) -> Bus Creator2/26
  HMI2.12/48(Request_driveoff) -> Bus Creator/48
  HMI2.12/131(IFC_LeLane_dy) -> Bus Creator3/27
  Bus Selector6/5 -> HMI2.12/79(ObjTypeP1)  "<ObjTypeP1>"
  HMI2.12/66(ACC_RiTgt_02_Dx) -> Bus Creator/66
  HMI2.12/139(IFC_Handsoffwarn) -> Bus Creator3/35
  HMI2.12/4(ACC_InterSysInfoDisp) -> Bus Creator/4
  HMI2.12/64(ACC_RiTargrt_02_Detn) -> Bus Creator/64
  HMI2.12/82(ACC_TgtObjVy) -> Bus Creator2/5
  Bus Creator4/1 -> HMI_IFC_FD5/1
  Bus Selector/17 -> HMI2.12/23(LDWState)  "<LDWSts>"
  HMI2.12/108(LCKResp) -> Bus Creator3/4
  Bus Selector5/2 -> HMI2.12/57(Camera_BlockageSts)  "<FCam_BlockageSts>"
  HMI2.12/22(HWASnvtySetResp) -> Bus Creator/22
  Bus Selector8/5 -> HMI2.12/93(ObjTypeP3)  "<ObjTypeP3>"
  Bus Selector3/6 -> HMI2.12/6(HWAAccControlSts)  "<HWAAccControlSts>"
  HMI2.12/71(Longctrl_DrvOFF_Req) -> Bus Creator1/1
  Bus Selector2/11 -> HMI2.12/69(ObjDYP0)  "<ObjDYP0>"
  HMI2.12/88(ACC_TgtObjCntAlive) -> Bus Creator2/11
  Bus Selector13/1 -> HMI2.12/120(L2dC0V)  "<dC0V>"
  HMI2.12/169(IFC_Line04_HeadingAngle) -> Bus Creator5/4
  HMI2.12/62(ACC_LeTgt_02_Typ) -> Bus Creator/62
  HMI2.12/60(ACC_LeTgt_02_Dy) -> Bus Creator/60
  HMI2.12/119(AESResp) -> Bus Creator3/15
  HMI2.12/121(LDW_LKA_Snvty) -> Bus Creator3/17
  HMI2.12/160(IFC_Roadedge01_CurvChange) -> Bus Creator4/19
  TOS_ACCP4/1 -> Bus Selector9/1
  Bus Selector/37 -> HMI2.12/43(TJA_FollowSts)  "<TJA_FollowSts>"
  HMI2.12/153(IFC_Line03_Type) -> Bus Creator4/12
  Bus Selector8/2 -> HMI2.12/90(dxP3)  "<dxP3>"
  HMI2.12/96(CurveDst) -> Bus Creator2/19
  HMI2.12/36(ACC_RiTgtTyp) -> Bus Creator/36
  HMI2.12/5(TJA_ICA_InterSysInfoDisp) -> Bus Creator/5
  HMI2.12/54(ACC_LeTgtfusion) -> Bus Creator/54
  Bus Selector3/5 -> HMI2.12/5(vSetBelowMin)  "<vSetBelowMin>"
  HMI2.12/161(IFC_Roadedge01_Type) -> Bus Creator4/20
  HMI2.12/123(IFC_HUTInterface) -> Bus Creator3/19
  HMI2.12/136(ESSintervention) -> Bus Creator3/32
  HMI2.12/21(ADAS_DriverInloop_Monitor) -> Bus Creator/21
  HMI2.12/186(ESSErrSts) -> HMI_ESSErrSts/1
  Bus Selector26/1 -> HMI2.12/169(LKASwtReq)  "<LKASwtReq>"
  Bus Selector/19 -> HMI2.12/25(LKAWarning)  "<LKAWarning>"
  HMI2.12/23(HWA_Lane_ChangeReq) -> Bus Creator/23
  RFM_LINE_L1/1 -> Bus Selector11/1
  Bus Selector22/2 -> HMI2.12/153(BridgeDistance)  "<f_bridge_distance>"
  HMI2.12/187(IDC_L2_EmgyLightReq) -> Bus Creator6/1
  Bus Selector22/1 -> HMI2.12/152(TunnelDistance)  "<f_toll_distance>"
  HMI2.12/29(ACC_PotentialTgtDx) -> Bus Creator/29
  Bus Creator6/1 -> HMI_IFC_FD3/1
  Bus Selector2/14 -> HMI2.12/72(ACCTgtObjCntAlive)  "<ACCTgtObjCntAlive>"
  HMI2.12/122(IFCCalibrationSts) -> Bus Creator3/18
  Bus Selector/24 -> HMI2.12/30(ISLActive)  "<ISLActive>"
  Bus Selector/41 -> HMI2.12/47(ACC_DrvrOffDisp)  "<ACC_DrvrOffDisp>"
  HMI2.12/45(ACC_RlvTgtDy) -> Bus Creator/45
  HMI2.12/46(Longctrl_HCUTrqReq_DVR) -> Bus Creator/46
  Bus Selector11/1 -> [L1LineExist]  "<bIsLineExist>"
  Bus Selector11/3 -> [L1C1]  "<dC1V>"
  Bus Selector11/4 -> [L1C2]  "<dC2V>"
  Bus Selector11/5 -> [L1C3]  "<dC3V>"
  Bus Selector12/1 -> [R1LineExist]  "<bIsLineExist>"
  Bus Selector12/3 -> [R1C1]  "<dC1V>"
  Bus Selector12/4 -> [R1C2]  "<dC2V>"
  Bus Selector12/5 -> [R1C3]  "<dC3V>"
  Bus Selector13/2 -> Terminator/1  "<dC1V>"
  Bus Selector13/3 -> Terminator1/1  "<dC2V>"
  Bus Selector13/4 -> Terminator2/1  "<dC3V>"
  Bus Selector13/8 -> HMI2.12/127(L2LineExist)  "<bIsLineExist>"
  Bus Selector14/8 -> HMI2.12/135(R2LineExist)  "<bIsLineExist>"
  Bus Selector14/2 -> Terminator4/1  "<dC1V>"
  Bus Selector14/3 -> Terminator5/1  "<dC2V>"
  Bus Selector14/4 -> Terminator6/1  "<dC3V>"
  [L1LineExist] -> HMI2.12/104("L1blsLineExist ")
  [R1LineExist] -> HMI2.12/112("R1blsLineExist ")
  [A1] -> HMI2.12/106(L1dC1V)
  [A2] -> HMI2.12/107(L1dC2V)
  [A3] -> HMI2.12/108(L1dC3V)
  [A2] -> HMI2.12/115(R1dC2V)
  [A1] -> HMI2.12/114(R1dC1V)
  [A3] -> HMI2.12/116(R1dC3V)
  [A2] -> HMI2.12/122(L2dC2V)
  [A1] -> HMI2.12/121(L2dC1V)
  [A3] -> HMI2.12/123(L2dC3V)
  [A2] -> HMI2.12/130(R2dC2V)
  [A1] -> HMI2.12/129(R2dC1V)
  [A3] -> HMI2.12/131(R2dC3V)
  Bus Selector15/2 -> HMI2.12/137(F_LBdC0V)  "<dC0V>"
  MATLAB Function1/3(A3) -> [A3]
  MATLAB Function1/2(A2) -> [A2]
  MATLAB Function1/1(A1) -> [A1]
  [R1C3] -> MATLAB Function1/8(Ri1C3)
  [R1C2] -> MATLAB Function1/7(Ri1C2)
  [R1C1] -> MATLAB Function1/6(Ri1C1)
  [L1C3] -> MATLAB Function1/5(Le1C3)
  [L1C2] -> MATLAB Function1/4(Le1C2)
  [L1C1] -> MATLAB Function1/3(Le1C1)
  [R1LineExist] -> MATLAB Function1/2(Ri1LineExist)
  [L1LineExist] -> MATLAB Function1/1(Le1LineExist)
  Bus Selector15/1 -> [LB_Exist]  "<bIsLineExist>"
  [LB_Exist] -> HMI2.12/136(F_LBblsLineExist)
  Bus Selector15/3 -> [LB_C1]  "<dC1V>"
  Bus Selector15/4 -> [LB_C2]  "<dC2V>"
  Bus Selector15/5 -> [LB_C3]  "<dC3V>"
  Bus Selector16/1 -> [RB_Exist]  "<bIsLineExist>"
  Bus Selector16/3 -> [RB_C1]  "<dC1V>"
  Bus Selector16/4 -> [RB_C2]  "<dC2V>"
  Bus Selector16/5 -> [RB_C3]  "<dC3V>"
  [LB_Exist] -> MATLAB Function1/9(LB_Exist)
  [LB_C1] -> MATLAB Function1/10(LB_C1)
  [LB_C3] -> MATLAB Function1/12(LB_C3)
  [LB_C2] -> MATLAB Function1/11(LB_C2)
  [RB_Exist] -> MATLAB Function1/13(RB_Exist)
  [RB_C3] -> MATLAB Function1/16(RB_C3)
  [RB_C2] -> MATLAB Function1/15(RB_C2)
  [RB_C1] -> MATLAB Function1/14(RB_C1)
  [A1] -> HMI2.12/138(F_LBdC1V)
  [A2] -> HMI2.12/139(F_LBdC2V)
  [A3] -> HMI2.12/140(F_LBdC3V)
  [A1] -> HMI2.12/146(F_RBdC1V)
  [A2] -> HMI2.12/147(F_RBdC2V)
  [A3] -> HMI2.12/148(F_RBdC3V)
  [RB_Exist] -> HMI2.12/144(F_RBblsLineExist)
  standstill/1 -> HMI2.12/172(standstill)
